simulink library "lib_S7RRRRRRR1_dynamics"  (Simulink 8.5)
settings: Solver=ode45  StartTime=0.0  StopTime=10.0  RelTol=1e-3
values from neighbouring files (symbols this model uses):
  MPV = t1    [S7RRRRRRR1_convert_par2_MPV_fixb.m]
undefined symbols (not defined in the file or in its folder): eulxyz2r, eulxyzD2omega, g_base, g_world, phi_base_t0, phiD_base_t0, pkin, q_t0, qD_t0
undefined symbols (not defined in the file): DynPar1, qJ_t0, qJD_t0, r_base_t0, rD_base_t0
libraries: lib_S7RRRRRRR1_dynamics x20, lib_transformations x8, lib_rigid_body_kinematics x6
settings Model: Creator=schappler  LastModifiedBy=schappler

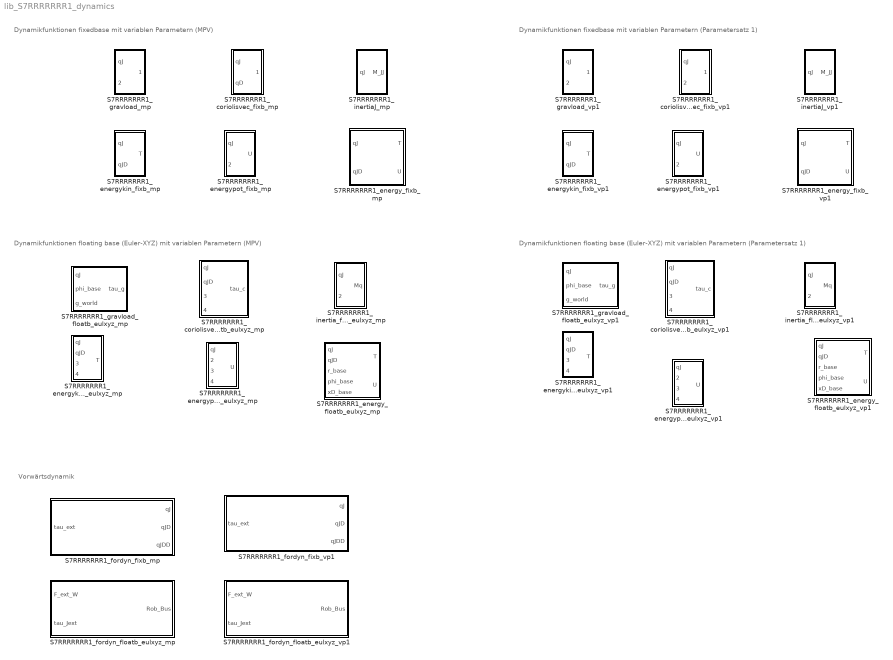
== system lib_S7RRRRRRR1_dynamics ==
  note: Vorwärtsdynamik
  note: Dynamikfunktionen fixedbase mit variablen Parametern (MPV)
  note: Dynamikfunktionen fixedbase mit variablen Parametern (Parametersatz 1)
  note: Dynamikfunktionen floating base (Euler-XYZ) mit variablen Parametern (Parametersatz 1)
  note: Dynamikfunktionen floating base (Euler-XYZ) mit variablen Parametern (MPV)
  S7RRRRRRR1_coriolisvec_fixb_mp : Subsystem  mask{pkin=pkin, MPV=MPV}
      mask prompts: pkin "Kinematik-Parameter"; MPV "Dynamik-Parameter (Minimalparametervektor fixed-base)"
      mask init:
      | NQJ=7;
  S7RRRRRRR1_coriolisvec_fixb_vp1 : Subsystem  mask{pkin=pkin, DynPar1=DynPar1}
      mask prompts: pkin "Kinematik-Parameter"; DynPar1 "Dynamik-Parameter (Parametersatz 1)"
      mask init:
      | NQJ=7;
      | m = DynPar1.m;
      | r_S = DynPar1.r_S;
      | I_S = DynPar1.I_S;
  S7RRRRRRR1_coriolisvec_floatb_eulxyz_mp : Subsystem  mask{pkin=pkin, MPV=MPV}
      mask prompts: pkin "Kinematik-Parameter"; MPV "Dynamik-Parameter (Minimalparametervektor floating-base)"
      mask init:
      | NQJ=7;
  S7RRRRRRR1_coriolisvec_floatb_eulxyz_vp1 : Subsystem  mask{pkin=pkin, DynPar1=DynPar1}
      mask prompts: pkin "Kinematik-Parameter"; DynPar1 "Dynamik-Parameter (Parametersatz 1)"
      mask init:
      | NQJ=7;
      | m = DynPar1.m;
      | r_S = DynPar1.r_S;
      | I_S = DynPar1.I_S;
  S7RRRRRRR1_energy_fixb_mp : Subsystem  mask{pkin=pkin, MPV=MPV, g_base=g_base}
      mask prompts: pkin "Kinematik-Parameter"; MPV "Dynamik-Parameter (Minimalparametervektor fixed-base)"; g_base "Gravitationsvektor im Basis-KS (g_base)"
      mask init:
      | NQJ=7;
  S7RRRRRRR1_energy_fixb_vp1 : Subsystem  mask{pkin=pkin, DynPar1=DynPar1, g_base=g_base}
      mask prompts: pkin "Kinematik-Parameter"; DynPar1 "Dynamik-Parameter (Parametersatz 1)"; g_base "Gravitationsvektor im Basis-KS (g_base)"
      mask init:
      | NQJ=7;
  S7RRRRRRR1_energy_floatb_eulxyz_mp : Subsystem  mask{pkin=pkin, MPV=MPV, g_world=g_world}
      mask prompts: pkin "Kinematik-Parameter"; MPV "Dynamik-Parameter (Minimalparametervektor floating-base)"; g_world "Gravitationsvektor im Welt-KS (g_world)"
      mask init:
      | NQJ=7;
  S7RRRRRRR1_energy_floatb_eulxyz_vp1 : Subsystem  mask{pkin=pkin, DynPar1=DynPar1, g_world=g_world}
      mask prompts: pkin "Kinematik-Parameter"; DynPar1 "Dynamik-Parameter (Parametersatz 1)"; g_world "Gravitationsvektor im Welt-KS (g_world)"
      mask init:
      | NQJ=7;
  S7RRRRRRR1_energykin_fixb_mp : Subsystem  mask{pkin=pkin, MPV=MPV}
      mask prompts: pkin "Kinematik-Parameter"; MPV "Dynamik-Parameter (Minimalparametervektor fixed-base)"
  S7RRRRRRR1_energykin_fixb_vp1 : Subsystem  mask{pkin=pkin, DynPar1=DynPar1}
      mask prompts: pkin "Kinematik-Parameter"; DynPar1 "Dynamik-Parameter (Parametersatz 1)"
      mask init:
      | NQJ=7;
      | m = DynPar1.m;
      | r_S = DynPar1.r_S;
      | I_S = DynPar1.I_S;
  S7RRRRRRR1_energykin_floatb_eulxyz_mp : Subsystem  mask{pkin=pkin, MPV=MPV}
      mask prompts: pkin "Kinematik-Parameter"; MPV "Dynamik-Parameter (Minimalparametervektor floating-base)"
      mask init:
      | NQJ=7;
  S7RRRRRRR1_energykin_floatb_eulxyz_vp1 : Subsystem  mask{pkin=pkin, DynPar1=DynPar1}
      mask prompts: pkin "Kinematik-Parameter"; DynPar1 "Dynamik-Parameter (Parametersatz 1)"
      mask init:
      | NQJ=7;
      | m = DynPar1.m;
      | r_S = DynPar1.r_S;
      | I_S = DynPar1.I_S;
  S7RRRRRRR1_energypot_fixb_mp : Subsystem  mask{pkin=pkin, MPV=MPV}
      mask prompts: pkin "Kinematik-Parameter"; MPV "Dynamik-Parameter (Minimalparametervektor fixed-base)"
      mask init:
      | NQJ=7;
  S7RRRRRRR1_energypot_fixb_vp1 : Subsystem  mask{pkin=pkin, DynPar1=DynPar1}
      mask prompts: pkin "Kinematik-Parameter"; DynPar1 "Dynamik-Parameter (Parametersatz 1)"
      mask init:
      | NQJ=7;
      | m = DynPar1.m;
      | r_S = DynPar1.r_S;
      | I_S = DynPar1.I_S;
  S7RRRRRRR1_energypot_floatb_eulxyz_mp : Subsystem  mask{pkin=pkin, MPV=MPV}
      mask prompts: pkin "Kinematik-Parameter"; MPV "Dynamik-Parameter (Minimalparametervektor floating-base)"
      mask init:
      | NQJ=7;
  S7RRRRRRR1_energypot_floatb_eulxyz_vp1 : Subsystem  mask{pkin=pkin, DynPar1=DynPar1}
      mask prompts: pkin "Kinematik-Parameter"; DynPar1 "Dynamik-Parameter (Parametersatz 1)"
      mask init:
      | NQJ=7;
      | m = DynPar1.m;
      | r_S = DynPar1.r_S;
      | I_S = DynPar1.I_S;
  S7RRRRRRR1_fordyn_fixb_mp : Subsystem  mask{q_t0=q_t0, qD_t0=qD_t0, g_base=g_base, pkin=pkin, MPV=MPV}
      mask prompts: q_t0 "q0 (initial pose)"; qD_t0 "qD0 (initial velocity)"; pkin "Kinematik-Parameter"; MPV "Dynamik-Parameter (Minimalparametervektor fixed-base)"
      mask init:
      | NQJ=7;
  S7RRRRRRR1_fordyn_fixb_vp1 : Subsystem  mask{q_t0=q_t0, qD_t0=qD_t0, g_base=g_base, pkin=pkin, DynPar1=DynPar1}
      mask prompts: q_t0 "q0 (initial pose)"; qD_t0 "qD0 (initial velocity)"; pkin "Kinematik-Parameter"; DynPar1 "Dynamik-Parameter (Parametersatz 1)"
      mask init:
      | NQJ=7;
  S7RRRRRRR1_fordyn_floatb_eulxyz_mp : Subsystem  mask{r_base_t0=r_base_t0, rD_base_t0=rD_base_t0, phi_base_t0=phi_base_t0, phiD_base_t0=phiD_base_t0, qJ_t0=qJ_t0, qJD_t0=qJD_t0, g_world=g_world, pkin=pkin, MPV=MPV}
      mask prompts: r_base_t0 "r_base_t0 (Basisposition im Welt-KS)"; qJ_t0 "q0 (initial pose)"; qJD_t0 "qD0 (initial velocity)"; pkin "Kinematik-Parameter"; MPV "Dynamik-Parameter (Minimalparametervektor floating-base)"
      mask init:
      | NQJ=7;
      mask Display:
      | port_label('input', 1, '_{(W)} F^{ext}', 'texmode', 'on')
      | port_label('input', 2, '\tau^{ext}_{J}', 'texmode', 'on')
      | port_label('output', 1, 'Rob_Bus')
  S7RRRRRRR1_fordyn_floatb_eulxyz_vp1 : Subsystem  mask{r_base_t0=r_base_t0, rD_base_t0=rD_base_t0, phi_base_t0=phi_base_t0, phiD_base_t0=phiD_base_t0, qJ_t0=qJ_t0, qJD_t0=qJD_t0, g_world=g_world, pkin=pkin, DynPar1=DynPar1}
      mask prompts: r_base_t0 "r_base_t0 (Basisposition im Welt-KS)"; qJ_t0 "q0 (initial pose)"; qJD_t0 "qD0 (initial velocity)"; pkin "Kinematik-Parameter"; DynPar1 "Dynamik-Parameter (Parametersatz 1)"
      mask init:
      | NQJ=7;
      mask Display:
      | port_label('input', 1, '_{(W)} F^{ext}', 'texmode', 'on')
      | port_label('input', 2, '\tau^{ext}_{J}', 'texmode', 'on')
      | port_label('output', 1, 'Rob_Bus')
  S7RRRRRRR1_gravload_floatb_eulxyz_mp : Subsystem  mask{pkin=pkin, MPV=MPV}
      mask prompts: pkin "Kinematik-Parameter"; MPV "Dynamik-Parameter (Minimalparametervektor floating-base)"
      mask init:
      | NQJ=7;
  S7RRRRRRR1_gravload_floatb_eulxyz_vp1 : Subsystem  mask{pkin=pkin, DynPar1=DynPar1}
      mask prompts: pkin "Kinematik-Parameter"; DynPar1 "Dynamik-Parameter (Parametersatz 1)"
      mask init:
      | NQJ=7;
      | m = DynPar1.m;
      | r_S = DynPar1.r_S;
      | I_S = DynPar1.I_S;
  S7RRRRRRR1_gravload_mp : Subsystem  mask{pkin=pkin, MPV=MPV}
      mask prompts: pkin "Kinematik-Parameter"; MPV "Dynamik-Parameter (Minimalparametervektor fixed-base)"
      mask init:
      | NQJ=7;
  S7RRRRRRR1_gravload_vp1 : Subsystem  mask{pkin=pkin, DynPar1=DynPar1}
      mask prompts: pkin "Kinematik-Parameter"; DynPar1 "Dynamik-Parameter (Parametersatz 1)"
      mask init:
      | NQJ=7;
      | m = DynPar1.m;
      | r_S = DynPar1.r_S;
      | I_S = DynPar1.I_S;
  S7RRRRRRR1_inertiaJ_mp : Subsystem  mask{pkin=pkin, MPV=MPV}
      mask prompts: pkin "Kinematik-Parameter"; MPV "Dynamik-Parameter (Minimalparametervektor fixed-base)"
      mask init:
      | NQJ=7;
  S7RRRRRRR1_inertiaJ_vp1 : Subsystem  mask{pkin=pkin, DynPar1=DynPar1}
      mask prompts: pkin "Kinematik-Parameter"; DynPar1 "Dynamik-Parameter (Parametersatz 1)"
      mask init:
      | NQJ=7;
      | m = DynPar1.m;
      | r_S = DynPar1.r_S;
      | I_S = DynPar1.I_S;
  S7RRRRRRR1_inertia_floatb_eulxyz_mp : Subsystem  mask{pkin=pkin, MPV=MPV}
      mask prompts: pkin "Kinematik-Parameter"; MPV "Dynamik-Parameter (Minimalparametervektor floating-base)"
      mask init:
      | NQJ=7;
  S7RRRRRRR1_inertia_floatb_eulxyz_vp1 : Subsystem  mask{pkin=pkin, DynPar1=DynPar1}
      mask prompts: pkin "Kinematik-Parameter"; DynPar1 "Dynamik-Parameter (Parametersatz 1)"
      mask init:
      | NQJ=7;
      | m = DynPar1.m;
      | r_S = DynPar1.r_S;
      | I_S = DynPar1.I_S;

== system lib_S7RRRRRRR1_dynamics/S7RRRRRRR1_coriolisvec_fixb_mp ==
  qJ : Inport  PortDimensions=NQJ
  qD : Inport  Port=2
  Constant5 : Constant  Value=MPV
  Constant6 : Constant  Value=pkin
  coriolisvec_fcn : MATLAB Function  TreatAsAtomicUnit=on
  tauJ_c : Outport  PortDimensions=NQJ
  wires:
  coriolisvec_fcn/1(taug) -> tauJ_c/1
  Constant6/1 -> coriolisvec_fcn/3(pkin)
  qD/1 -> coriolisvec_fcn/2(qD)
  qJ/1 -> coriolisvec_fcn/1(q)
  Constant5/1 -> coriolisvec_fcn/4(MPV)

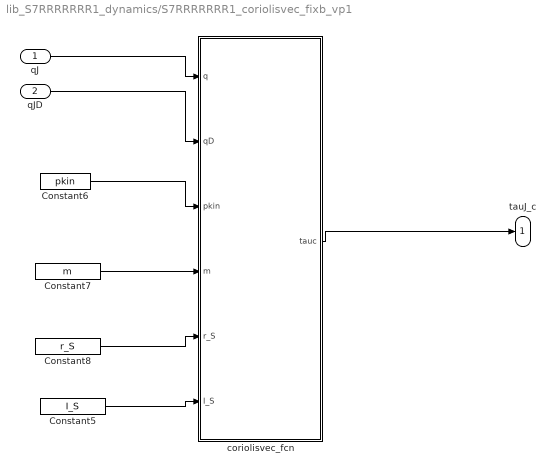
== system lib_S7RRRRRRR1_dynamics/S7RRRRRRR1_coriolisvec_fixb_vp1 ==
  qJ : Inport  PortDimensions=NQJ
  qJD : Inport  Port=2  PortDimensions=NQJ
  Constant5 : Constant  Value=I_S
  Constant6 : Constant  Value=pkin
  Constant7 : Constant  Value=m
  Constant8 : Constant  Value=r_S
  coriolisvec_fcn : MATLAB Function  TreatAsAtomicUnit=on
  tauJ_c : Outport  PortDimensions=NQJ
  wires:
  coriolisvec_fcn/1(tauc) -> tauJ_c/1
  Constant6/1 -> coriolisvec_fcn/3(pkin)
  qJD/1 -> coriolisvec_fcn/2(qD)
  qJ/1 -> coriolisvec_fcn/1(q)
  Constant7/1 -> coriolisvec_fcn/4(m)
  Constant8/1 -> coriolisvec_fcn/5(r_S)
  Constant5/1 -> coriolisvec_fcn/6(I_S)

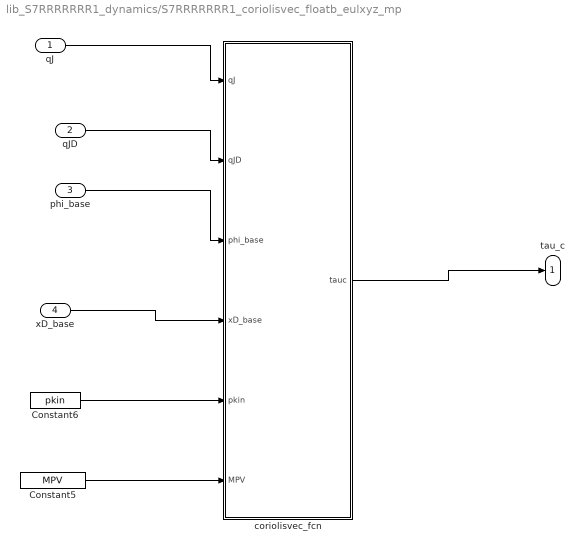
== system lib_S7RRRRRRR1_dynamics/S7RRRRRRR1_coriolisvec_floatb_eulxyz_mp ==
  qJ : Inport  PortDimensions=NQJ
  qJD : Inport  Port=2  PortDimensions=NQJ
  phi_base : Inport  Port=3  PortDimensions=3
  xD_base : Inport  Port=4  PortDimensions=6
  Constant5 : Constant  Value=MPV
  Constant6 : Constant  Value=pkin
  coriolisvec_fcn : MATLAB Function  TreatAsAtomicUnit=on
  tau_c : Outport  PortDimensions=6+NQJ
  wires:
  coriolisvec_fcn/1(tauc) -> tau_c/1
  Constant6/1 -> coriolisvec_fcn/5(pkin)
  qJD/1 -> coriolisvec_fcn/2(qJD)
  qJ/1 -> coriolisvec_fcn/1(qJ)
  Constant5/1 -> coriolisvec_fcn/6(MPV)
  phi_base/1 -> coriolisvec_fcn/3(phi_base)
  xD_base/1 -> coriolisvec_fcn/4(xD_base)

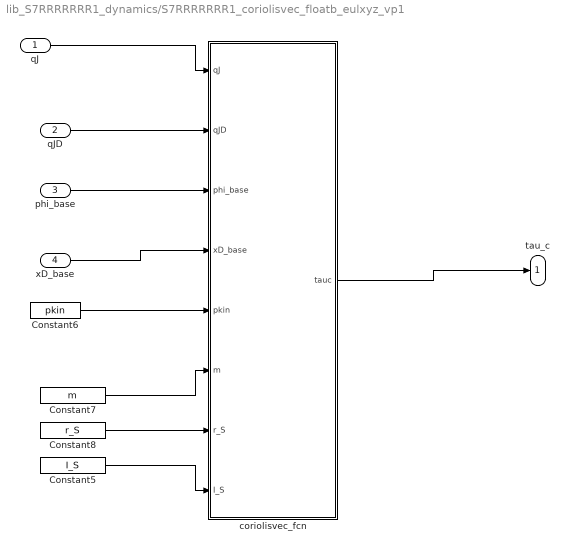
== system lib_S7RRRRRRR1_dynamics/S7RRRRRRR1_coriolisvec_floatb_eulxyz_vp1 ==
  qJ : Inport  PortDimensions=NQJ
  qJD : Inport  Port=2  PortDimensions=NQJ
  phi_base : Inport  Port=3  PortDimensions=3
  xD_base : Inport  Port=4  PortDimensions=6
  Constant5 : Constant  Value=I_S
  Constant6 : Constant  Value=pkin
  Constant7 : Constant  Value=m
  Constant8 : Constant  Value=r_S
  coriolisvec_fcn : MATLAB Function  TreatAsAtomicUnit=on
  tau_c : Outport  PortDimensions=6+NQJ
  wires:
  coriolisvec_fcn/1(tauc) -> tau_c/1
  Constant6/1 -> coriolisvec_fcn/5(pkin)
  qJD/1 -> coriolisvec_fcn/2(qJD)
  qJ/1 -> coriolisvec_fcn/1(qJ)
  Constant7/1 -> coriolisvec_fcn/6(m)
  Constant8/1 -> coriolisvec_fcn/7(r_S)
  Constant5/1 -> coriolisvec_fcn/8(I_S)
  phi_base/1 -> coriolisvec_fcn/3(phi_base)
  xD_base/1 -> coriolisvec_fcn/4(xD_base)

== system lib_S7RRRRRRR1_dynamics/S7RRRRRRR1_energy_fixb_mp ==
  qJ : Inport  PortDimensions=NQJ
  qJD : Inport  Port=2  PortDimensions=NQJ
  Constant : Constant  Value=g_base
  S7RRRRRRR1_energykin_fixb_mp : lib_S7RRRRRRR1_dynamics/S7RRRRRRR1_energykin_fixb_mp  pkin=pkin  MPV=MPV
  S7RRRRRRR1_energypot_fixb_mp : lib_S7RRRRRRR1_dynamics/S7RRRRRRR1_energypot_fixb_mp  pkin=pkin  MPV=MPV
  T : Outport  PortDimensions=1
  U : Outport  Port=2  PortDimensions=1
  wires:
  Constant/1 -> S7RRRRRRR1_energypot_fixb_mp/2
  qJD/1 -> S7RRRRRRR1_energykin_fixb_mp/2
  qJ/1 -> S7RRRRRRR1_energypot_fixb_mp/1, S7RRRRRRR1_energykin_fixb_mp/1
  S7RRRRRRR1_energypot_fixb_mp/1 -> U/1
  S7RRRRRRR1_energykin_fixb_mp/1 -> T/1

== system lib_S7RRRRRRR1_dynamics/S7RRRRRRR1_energy_fixb_vp1 ==
  qJ : Inport  PortDimensions=NQJ
  qJD : Inport  Port=2  PortDimensions=NQJ
  Constant : Constant  Value=g_base
  S7RRRRRRR1_energykin_fixb : lib_S7RRRRRRR1_dynamics/S7RRRRRRR1_energykin_fixb_vp1  pkin=pkin  DynPar1=DynPar1
  S7RRRRRRR1_energypot_fixb : lib_S7RRRRRRR1_dynamics/S7RRRRRRR1_energypot_fixb_vp1  pkin=pkin  DynPar1=DynPar1
  T : Outport  PortDimensions=1
  U : Outport  Port=2  PortDimensions=1
  wires:
  Constant/1 -> S7RRRRRRR1_energypot_fixb/2
  qJD/1 -> S7RRRRRRR1_energykin_fixb/2
  qJ/1 -> S7RRRRRRR1_energypot_fixb/1, S7RRRRRRR1_energykin_fixb/1
  S7RRRRRRR1_energypot_fixb/1 -> U/1
  S7RRRRRRR1_energykin_fixb/1 -> T/1

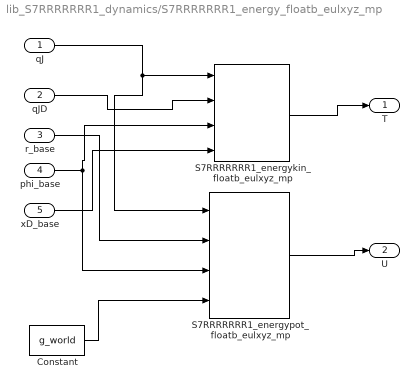
== system lib_S7RRRRRRR1_dynamics/S7RRRRRRR1_energy_floatb_eulxyz_mp ==
  qJ : Inport  PortDimensions=NQJ
  qJD : Inport  Port=2  PortDimensions=NQJ
  r_base : Inport  Port=3  PortDimensions=3
  phi_base : Inport  Port=4  PortDimensions=3
  xD_base : Inport  Port=5  PortDimensions=6
  Constant : Constant  Value=g_world
  S7RRRRRRR1_energykin_floatb_eulxyz_mp : lib_S7RRRRRRR1_dynamics/S7RRRRRRR1_energykin_floatb_eulxyz_mp  pkin=pkin  MPV=MPV
  S7RRRRRRR1_energypot_floatb_eulxyz_mp : lib_S7RRRRRRR1_dynamics/S7RRRRRRR1_energypot_floatb_eulxyz_mp  pkin=pkin  MPV=MPV
  T : Outport
  U : Outport  Port=2
  wires:
  Constant/1 -> S7RRRRRRR1_energypot_floatb_eulxyz_mp/4
  qJD/1 -> S7RRRRRRR1_energykin_floatb_eulxyz_mp/2
  qJ/1 -> S7RRRRRRR1_energypot_floatb_eulxyz_mp/1, S7RRRRRRR1_energykin_floatb_eulxyz_mp/1
  S7RRRRRRR1_energypot_floatb_eulxyz_mp/1 -> U/1
  S7RRRRRRR1_energykin_floatb_eulxyz_mp/1 -> T/1
  phi_base/1 -> S7RRRRRRR1_energypot_floatb_eulxyz_mp/3, S7RRRRRRR1_energykin_floatb_eulxyz_mp/3
  r_base/1 -> S7RRRRRRR1_energypot_floatb_eulxyz_mp/2
  xD_base/1 -> S7RRRRRRR1_energykin_floatb_eulxyz_mp/4

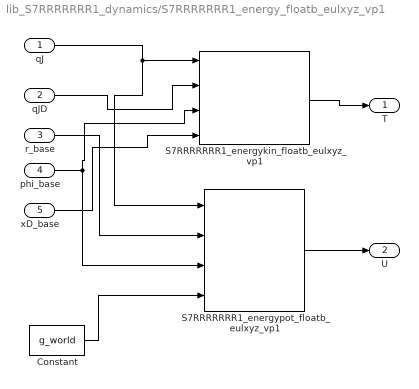
== system lib_S7RRRRRRR1_dynamics/S7RRRRRRR1_energy_floatb_eulxyz_vp1 ==
  qJ : Inport  PortDimensions=NQJ
  qJD : Inport  Port=2  PortDimensions=NQJ
  r_base : Inport  Port=3  PortDimensions=3
  phi_base : Inport  Port=4  PortDimensions=3
  xD_base : Inport  Port=5  PortDimensions=6
  Constant : Constant  Value=g_world
  S7RRRRRRR1_energykin_floatb_eulxyz_vp1 : lib_S7RRRRRRR1_dynamics/S7RRRRRRR1_energykin_floatb_eulxyz_vp1  pkin=pkin  DynPar1=DynPar1
  S7RRRRRRR1_energypot_floatb_eulxyz_vp1 : lib_S7RRRRRRR1_dynamics/S7RRRRRRR1_energypot_floatb_eulxyz_vp1  pkin=pkin  DynPar1=DynPar1
  T : Outport
  U : Outport  Port=2
  wires:
  Constant/1 -> S7RRRRRRR1_energypot_floatb_eulxyz_vp1/4
  qJD/1 -> S7RRRRRRR1_energykin_floatb_eulxyz_vp1/2
  qJ/1 -> S7RRRRRRR1_energypot_floatb_eulxyz_vp1/1, S7RRRRRRR1_energykin_floatb_eulxyz_vp1/1
  S7RRRRRRR1_energypot_floatb_eulxyz_vp1/1 -> U/1
  S7RRRRRRR1_energykin_floatb_eulxyz_vp1/1 -> T/1
  phi_base/1 -> S7RRRRRRR1_energykin_floatb_eulxyz_vp1/3, S7RRRRRRR1_energypot_floatb_eulxyz_vp1/3
  r_base/1 -> S7RRRRRRR1_energypot_floatb_eulxyz_vp1/2
  xD_base/1 -> S7RRRRRRR1_energykin_floatb_eulxyz_vp1/4

== system lib_S7RRRRRRR1_dynamics/S7RRRRRRR1_energykin_fixb_mp ==
  qJ : Inport  PortDimensions=NQJ
  qJD : Inport  Port=2  PortDimensions=NQJ
  Constant5 : Constant  Value=MPV
  Constant6 : Constant  Value=pkin
  energykin_fcn : MATLAB Function  TreatAsAtomicUnit=on
  T : Outport  PortDimensions=1
  wires:
  energykin_fcn/1(T) -> T/1
  Constant6/1 -> energykin_fcn/3(pkin)
  qJD/1 -> energykin_fcn/2(qD)
  qJ/1 -> energykin_fcn/1(q)
  Constant5/1 -> energykin_fcn/4(MPV)

== system lib_S7RRRRRRR1_dynamics/S7RRRRRRR1_energykin_fixb_vp1 ==
  qJ : Inport  PortDimensions=NQJ
  qJD : Inport  Port=2  PortDimensions=NQJ
  Constant5 : Constant  Value=I_S
  Constant6 : Constant  Value=pkin
  Constant7 : Constant  Value=m
  Constant8 : Constant  Value=r_S
  MATLAB Function : MATLAB Function  TreatAsAtomicUnit=on
  T : Outport
  wires:
  MATLAB Function/1(T) -> T/1
  Constant6/1 -> MATLAB Function/3(pkin)
  qJD/1 -> MATLAB Function/2(qD)
  qJ/1 -> MATLAB Function/1(q)
  Constant7/1 -> MATLAB Function/4(m)
  Constant8/1 -> MATLAB Function/5(r_S)
  Constant5/1 -> MATLAB Function/6(I_S)

== system lib_S7RRRRRRR1_dynamics/S7RRRRRRR1_energykin_floatb_eulxyz_mp ==
  qJ : Inport  PortDimensions=NQJ
  qJD : Inport  Port=2  PortDimensions=NQJ
  phi_base : Inport  Port=3  PortDimensions=3
  xD_base : Inport  Port=4  PortDimensions=6
  Constant1 : Constant  Value=MPV
  Constant6 : Constant  Value=pkin
  MATLAB Function : MATLAB Function  TreatAsAtomicUnit=on
  T : Outport  PortDimensions=1
  wires:
  MATLAB Function/1(T) -> T/1
  Constant6/1 -> MATLAB Function/5(pkin)
  qJD/1 -> MATLAB Function/2(qD)
  qJ/1 -> MATLAB Function/1(qJ)
  Constant1/1 -> MATLAB Function/6(MPV)
  phi_base/1 -> MATLAB Function/3(phi_base)
  xD_base/1 -> MATLAB Function/4(xD_base)

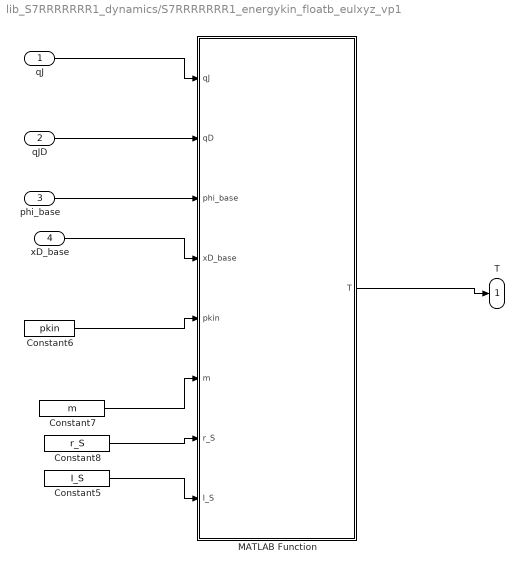
== system lib_S7RRRRRRR1_dynamics/S7RRRRRRR1_energykin_floatb_eulxyz_vp1 ==
  qJ : Inport  PortDimensions=NQJ
  qJD : Inport  Port=2  PortDimensions=NQJ
  phi_base : Inport  Port=3  PortDimensions=3
  xD_base : Inport  Port=4  PortDimensions=6
  Constant5 : Constant  Value=I_S
  Constant6 : Constant  Value=pkin
  Constant7 : Constant  Value=m
  Constant8 : Constant  Value=r_S
  MATLAB Function : MATLAB Function  TreatAsAtomicUnit=on
  T : Outport  PortDimensions=1
  wires:
  MATLAB Function/1(T) -> T/1
  Constant6/1 -> MATLAB Function/5(pkin)
  qJD/1 -> MATLAB Function/2(qD)
  qJ/1 -> MATLAB Function/1(qJ)
  Constant7/1 -> MATLAB Function/6(m)
  Constant8/1 -> MATLAB Function/7(r_S)
  Constant5/1 -> MATLAB Function/8(I_S)
  phi_base/1 -> MATLAB Function/3(phi_base)
  xD_base/1 -> MATLAB Function/4(xD_base)

== system lib_S7RRRRRRR1_dynamics/S7RRRRRRR1_energypot_fixb_mp ==
  qJ : Inport  PortDimensions=NQJ
  g_base : Inport  Port=2
  Constant5 : Constant  Value=MPV
  Constant6 : Constant  Value=pkin
  energypot_fcn : MATLAB Function  TreatAsAtomicUnit=on
  U : Outport  PortDimensions=1
  wires:
  energypot_fcn/1(T) -> U/1
  Constant6/1 -> energypot_fcn/3(pkin)
  g_base/1 -> energypot_fcn/2(g_base)
  qJ/1 -> energypot_fcn/1(q)
  Constant5/1 -> energypot_fcn/4(MPV)

== system lib_S7RRRRRRR1_dynamics/S7RRRRRRR1_energypot_fixb_vp1 ==
  qJ : Inport  PortDimensions=NQJ
  g_base : Inport  Port=2  PortDimensions=3
  Constant6 : Constant  Value=pkin
  Constant7 : Constant  Value=m
  Constant8 : Constant  Value=r_S
  MATLAB Function : MATLAB Function  TreatAsAtomicUnit=on
  U : Outport
  wires:
  MATLAB Function/1(U) -> U/1
  Constant6/1 -> MATLAB Function/3(pkin)
  g_base/1 -> MATLAB Function/2(g_base)
  qJ/1 -> MATLAB Function/1(q)
  Constant7/1 -> MATLAB Function/4(m)
  Constant8/1 -> MATLAB Function/5(r_S)

== system lib_S7RRRRRRR1_dynamics/S7RRRRRRR1_energypot_floatb_eulxyz_mp ==
  qJ : Inport  PortDimensions=NQJ
  r_base : Inport  Port=2  PortDimensions=3
  phi_base : Inport  Port=3  PortDimensions=3
  g_world : Inport  Port=4  PortDimensions=3
  Constant5 : Constant  Value=MPV
  Constant6 : Constant  Value=pkin
  MATLAB Function : MATLAB Function  TreatAsAtomicUnit=on
  U : Outport
  wires:
  MATLAB Function/1(U) -> U/1
  Constant6/1 -> MATLAB Function/5(pkin)
  g_world/1 -> MATLAB Function/4(g_world)
  qJ/1 -> MATLAB Function/1(qJ)
  r_base/1 -> MATLAB Function/2(r_base)
  phi_base/1 -> MATLAB Function/3(phi_base)
  Constant5/1 -> MATLAB Function/6(MPV)

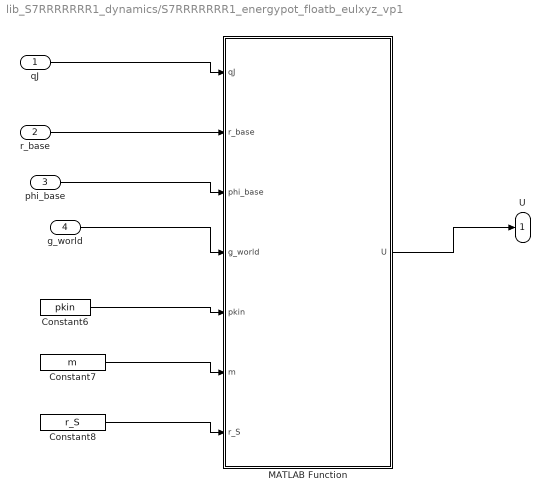
== system lib_S7RRRRRRR1_dynamics/S7RRRRRRR1_energypot_floatb_eulxyz_vp1 ==
  qJ : Inport  PortDimensions=NQJ
  r_base : Inport  Port=2  PortDimensions=3
  phi_base : Inport  Port=3  PortDimensions=3
  g_world : Inport  Port=4  PortDimensions=3
  Constant6 : Constant  Value=pkin
  Constant7 : Constant  Value=m
  Constant8 : Constant  Value=r_S
  MATLAB Function : MATLAB Function  TreatAsAtomicUnit=on
  U : Outport
  wires:
  MATLAB Function/1(U) -> U/1
  Constant6/1 -> MATLAB Function/5(pkin)
  g_world/1 -> MATLAB Function/4(g_world)
  qJ/1 -> MATLAB Function/1(qJ)
  Constant7/1 -> MATLAB Function/6(m)
  Constant8/1 -> MATLAB Function/7(r_S)
  r_base/1 -> MATLAB Function/2(r_base)
  phi_base/1 -> MATLAB Function/3(phi_base)

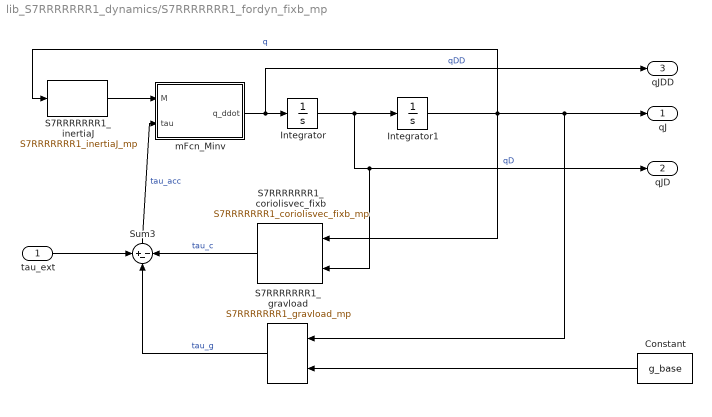
== system lib_S7RRRRRRR1_dynamics/S7RRRRRRR1_fordyn_fixb_mp ==
  "tau_ext " : Inport  PortDimensions=NQJ
  Constant : Constant  Value=g_base
  Integrator : Integrator  InitialCondition=qD_t0
  Integrator1 : Integrator  InitialCondition=q_t0
  Sum3 : Sum  Inputs=+--
  S7RRRRRRR1_coriolisvec_fixb : lib_S7RRRRRRR1_dynamics/S7RRRRRRR1_coriolisvec_fixb_mp  pkin=pkin  MPV=MPV
  S7RRRRRRR1_gravload : lib_S7RRRRRRR1_dynamics/S7RRRRRRR1_gravload_mp  pkin=pkin  MPV=MPV
  S7RRRRRRR1_inertiaJ : lib_S7RRRRRRR1_dynamics/S7RRRRRRR1_inertiaJ_mp  pkin=pkin  MPV=MPV
  mFcn_Minv : MATLAB Function  TreatAsAtomicUnit=on
  qJ : Outport  PortDimensions=NQJ
  qJD : Outport  Port=2  PortDimensions=NQJ
  qJDD : Outport  Port=3  PortDimensions=NQJ
  wires:
  S7RRRRRRR1_gravload/1 -> Sum3/2  "tau_g"
  Integrator1/1 -> S7RRRRRRR1_coriolisvec_fixb/1, S7RRRRRRR1_inertiaJ/1, S7RRRRRRR1_gravload/1, qJ/1  "q"
  mFcn_Minv/1(q_ddot) -> qJDD/1, Integrator/1  "qDD"
  S7RRRRRRR1_coriolisvec_fixb/1 -> Sum3/3  "tau_c"
  "tau_ext "/1 -> Sum3/1
  Integrator/1 -> S7RRRRRRR1_coriolisvec_fixb/2, qJD/1, Integrator1/1  "qD"
  Sum3/1 -> mFcn_Minv/2(tau)  "tau_acc"
  S7RRRRRRR1_inertiaJ/1 -> mFcn_Minv/1(M)
  Constant/1 -> S7RRRRRRR1_gravload/2

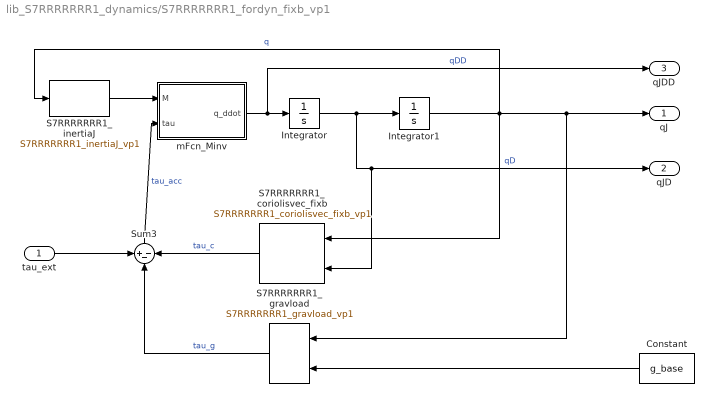
== system lib_S7RRRRRRR1_dynamics/S7RRRRRRR1_fordyn_fixb_vp1 ==
  "tau_ext " : Inport  PortDimensions=NQJ
  Constant : Constant  Value=g_base
  Integrator : Integrator  InitialCondition=qD_t0
  Integrator1 : Integrator  InitialCondition=q_t0
  Sum3 : Sum  Inputs=+--
  S7RRRRRRR1_coriolisvec_fixb : lib_S7RRRRRRR1_dynamics/S7RRRRRRR1_coriolisvec_fixb_vp1  pkin=pkin  DynPar1=DynPar1
  S7RRRRRRR1_gravload : lib_S7RRRRRRR1_dynamics/S7RRRRRRR1_gravload_vp1  pkin=pkin  DynPar1=DynPar1
  S7RRRRRRR1_inertiaJ : lib_S7RRRRRRR1_dynamics/S7RRRRRRR1_inertiaJ_vp1  pkin=pkin  DynPar1=DynPar1
  mFcn_Minv : MATLAB Function  TreatAsAtomicUnit=on
  qJ : Outport  PortDimensions=NQJ
  qJD : Outport  Port=2  PortDimensions=NQJ
  qJDD : Outport  Port=3  PortDimensions=NQJ
  wires:
  S7RRRRRRR1_gravload/1 -> Sum3/2  "tau_g"
  Integrator1/1 -> S7RRRRRRR1_coriolisvec_fixb/1, S7RRRRRRR1_inertiaJ/1, S7RRRRRRR1_gravload/1, qJ/1  "q"
  mFcn_Minv/1(q_ddot) -> qJDD/1, Integrator/1  "qDD"
  S7RRRRRRR1_coriolisvec_fixb/1 -> Sum3/3  "tau_c"
  "tau_ext "/1 -> Sum3/1
  Integrator/1 -> S7RRRRRRR1_coriolisvec_fixb/2, qJD/1, Integrator1/1  "qD"
  Sum3/1 -> mFcn_Minv/2(tau)  "tau_acc"
  S7RRRRRRR1_inertiaJ/1 -> mFcn_Minv/1(M)
  Constant/1 -> S7RRRRRRR1_gravload/2

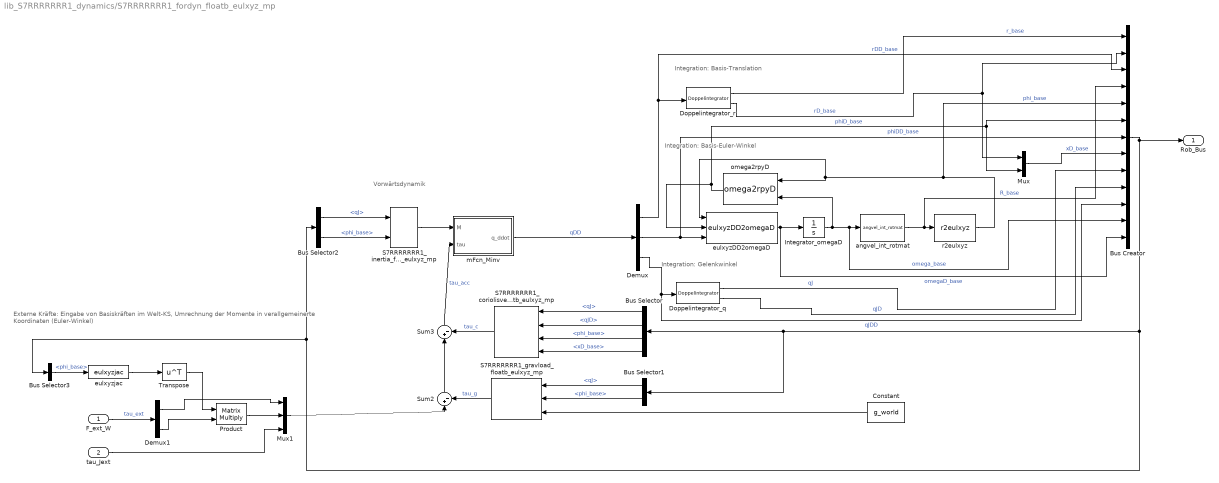
== system lib_S7RRRRRRR1_dynamics/S7RRRRRRR1_fordyn_floatb_eulxyz_mp ==
  note: Integration: Basis-Translation
  note: Integration: Gelenkwinkel
  note: Vorwärtsdynamik
  note: Integration: Basis-Euler-Winkel
  note: Externe Kräfte: Eingabe von Basiskräften im Welt-KS, Umrechnung der Momente
      | in verallgemeinerte Koordinaten (Euler-Winkel)
  F_ext_W : Inport  PortDimensions=6
  tau_Jext : Inport  Port=2  PortDimensions=NQJ
  Bus Creator : BusCreator  Inputs=13
  Bus Selector : BusSelector  OutputSignals=qJ,qJD,phi_base,xD_base
  Bus Selector1 : BusSelector  OutputSignals=qJ,phi_base
  Bus Selector2 : BusSelector  OutputSignals=qJ,phi_base
  Bus Selector3 : BusSelector  OutputSignals=phi_base
  Constant : Constant  Value=g_world
  Demux : Demux  Outputs=[3 3 NQJ]
  Demux1 : Demux  Outputs=[3 3]
  Doppelintegrator_q : lib_rigid_body_kinematics/Doppelintegrator  r0=qJ_t0  rD0=qJD_t0  Name_v='q'
  Doppelintegrator_r : lib_rigid_body_kinematics/Doppelintegrator  r0=r_base_t0  rD0=rD_base_t0  Name_v='r'
  Integrator_omegaD : Integrator  InitialCondition=eulxyzD2omega(phi_base_t0, phiD_base_t0)
  Mux : Mux  Inputs=2
  Mux1 : Mux  Inputs=[3 3 NQJ]
  Product : Product  Multiplication=Matrix(*)
  r2eulxyz : lib_transformations/r2eulxyz
  Sum2 : Sum  Inputs=|+-
  Sum3 : Sum  Inputs=|+-
  Transpose : Math  Operator=transpose  SaturateOnIntegerOverflow=on
  angvel_int_rotmat : lib_rigid_body_kinematics/angvel_int_rotmat  R_0E_t0=eulxyz2r(phi_base_t0)
  eulxyzjac : lib_transformations/eulxyzjac
  S7RRRRRRR1_coriolisvec_floatb_eulxyz_mp : lib_S7RRRRRRR1_dynamics/S7RRRRRRR1_coriolisvec_floatb_eulxyz_mp  pkin=pkin  MPV=MPV
  S7RRRRRRR1_gravload_floatb_eulxyz_mp : lib_S7RRRRRRR1_dynamics/S7RRRRRRR1_gravload_floatb_eulxyz_mp  pkin=pkin  MPV=MPV
  S7RRRRRRR1_inertia_floatb_eulxyz_mp : lib_S7RRRRRRR1_dynamics/S7RRRRRRR1_inertia_floatb_eulxyz_mp  pkin=pkin  MPV=MPV
  mFcn_Minv : MATLAB Function  TreatAsAtomicUnit=on
  omega2rpyD : lib_transformations/omega2rpyD
  eulxyzDD2omegaD : lib_transformations/eulxyzDD2omegaD
  Rob_Bus : Outport
  wires:
  Constant/1 -> S7RRRRRRR1_gravload_floatb_eulxyz_mp/3
  F_ext_W/1 -> Demux1/1  "tau_ext"
  S7RRRRRRR1_inertia_floatb_eulxyz_mp/1 -> mFcn_Minv/1(M)
  Sum3/1 -> mFcn_Minv/2(tau)  "tau_acc"
  S7RRRRRRR1_coriolisvec_floatb_eulxyz_mp/1 -> Sum3/2  "tau_c"
  Sum2/1 -> Sum3/1
  mFcn_Minv/1(q_ddot) -> Demux/1  "qDD"
  S7RRRRRRR1_gravload_floatb_eulxyz_mp/1 -> Sum2/2  "tau_g"
  Demux/1 -> Doppelintegrator_r/1, Bus Creator/3  "rDD_base"
  Demux/3 -> Bus Creator/11, Doppelintegrator_q/1  "qJDD"
  eulxyzDD2omegaD/1 -> Bus Creator/13, Integrator_omegaD/1  "omegaD_base"
  Integrator_omegaD/1 -> Bus Creator/12, angvel_int_rotmat/1, omega2rpyD/2  "omega_base"
  Demux/2 -> Bus Creator/7, eulxyzDD2omegaD/3  "phiDD_base"
  angvel_int_rotmat/1 -> Bus Creator/4, r2eulxyz/1  "R_base"
  r2eulxyz/1 -> Bus Creator/5, eulxyzDD2omegaD/1, omega2rpyD/1  "phi_base"
  omega2rpyD/1 -> eulxyzDD2omegaD/2, Mux/2, Bus Creator/6  "phiD_base"
  Doppelintegrator_r/1 -> Bus Creator/1  "r_base"
  Doppelintegrator_r/2 -> Mux/1, Bus Creator/2  "rD_base"
  Mux/1 -> Bus Creator/8  "xD_base"
  Doppelintegrator_q/1 -> Bus Creator/9  "qJ"
  Doppelintegrator_q/2 -> Bus Creator/10  "qJD"
  Bus Selector/4 -> S7RRRRRRR1_coriolisvec_floatb_eulxyz_mp/4  "<xD_base>"
  Bus Selector/3 -> S7RRRRRRR1_coriolisvec_floatb_eulxyz_mp/3  "<phi_base>"
  Bus Selector/2 -> S7RRRRRRR1_coriolisvec_floatb_eulxyz_mp/2  "<qJD>"
  Bus Selector/1 -> S7RRRRRRR1_coriolisvec_floatb_eulxyz_mp/1  "<qJ>"
  Bus Selector1/1 -> S7RRRRRRR1_gravload_floatb_eulxyz_mp/1  "<qJ>"
  Bus Selector1/2 -> S7RRRRRRR1_gravload_floatb_eulxyz_mp/2  "<phi_base>"
  Bus Selector2/1 -> S7RRRRRRR1_inertia_floatb_eulxyz_mp/1  "<qJ>"
  Bus Selector2/2 -> S7RRRRRRR1_inertia_floatb_eulxyz_mp/2  "<phi_base>"
  Bus Creator/1 -> Bus Selector2/1, Bus Selector3/1, Bus Selector1/1, Bus Selector/1, Rob_Bus/1
  Demux1/2 -> Product/2
  Bus Selector3/1 -> eulxyzjac/1  "<phi_base>"
  eulxyzjac/1 -> Transpose/1
  Product/1 -> Mux1/2
  Transpose/1 -> Product/1
  Demux1/1 -> Mux1/1
  tau_Jext/1 -> Mux1/3
  Mux1/1 -> Sum2/1

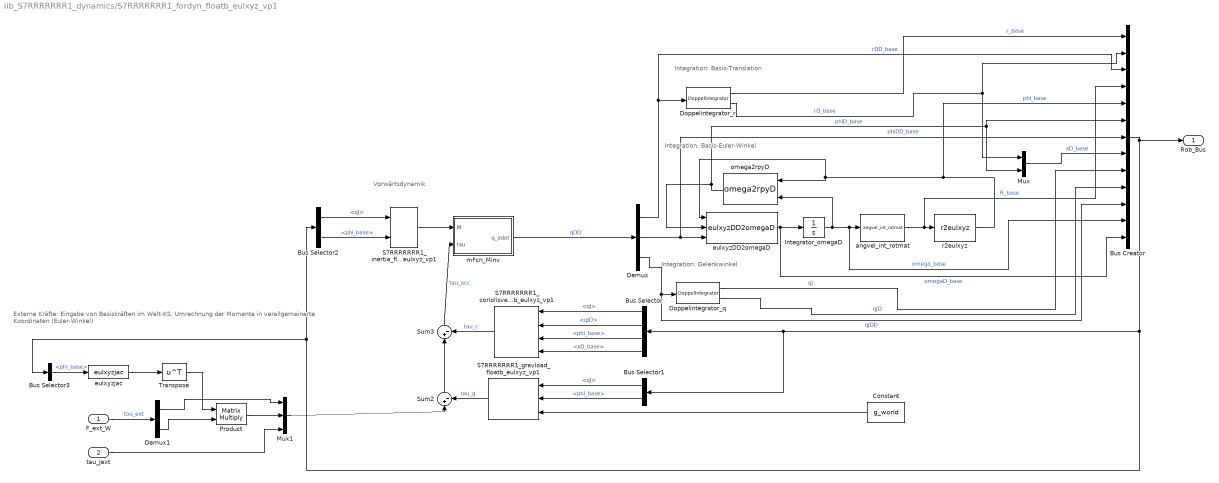
== system lib_S7RRRRRRR1_dynamics/S7RRRRRRR1_fordyn_floatb_eulxyz_vp1 ==
  note: Integration: Basis-Translation
  note: Integration: Gelenkwinkel
  note: Vorwärtsdynamik
  note: Integration: Basis-Euler-Winkel
  note: Externe Kräfte: Eingabe von Basiskräften im Welt-KS, Umrechnung der Momente
      | in verallgemeinerte Koordinaten (Euler-Winkel)
  F_ext_W : Inport  PortDimensions=6
  tau_Jext : Inport  Port=2  PortDimensions=NQJ
  Bus Creator : BusCreator  Inputs=13
  Bus Selector : BusSelector  OutputSignals=qJ,qJD,phi_base,xD_base
  Bus Selector1 : BusSelector  OutputSignals=qJ,phi_base
  Bus Selector2 : BusSelector  OutputSignals=qJ,phi_base
  Bus Selector3 : BusSelector  OutputSignals=phi_base
  Constant : Constant  Value=g_world
  Demux : Demux  Outputs=[3 3 NQJ]
  Demux1 : Demux  Outputs=[3 3]
  Doppelintegrator_q : lib_rigid_body_kinematics/Doppelintegrator  r0=qJ_t0  rD0=qJD_t0  Name_v='q'
  Doppelintegrator_r : lib_rigid_body_kinematics/Doppelintegrator  r0=r_base_t0  rD0=rD_base_t0  Name_v='r'
  Integrator_omegaD : Integrator  InitialCondition=eulxyzD2omega(phi_base_t0, phiD_base_t0)
  Mux : Mux  Inputs=2
  Mux1 : Mux  Inputs=[3 3 NQJ]
  Product : Product  Multiplication=Matrix(*)
  r2eulxyz : lib_transformations/r2eulxyz
  Sum2 : Sum  Inputs=|+-
  Sum3 : Sum  Inputs=|+-
  Transpose : Math  Operator=transpose  SaturateOnIntegerOverflow=on
  angvel_int_rotmat : lib_rigid_body_kinematics/angvel_int_rotmat  R_0E_t0=eulxyz2r(phi_base_t0)
  eulxyzjac : lib_transformations/eulxyzjac
  S7RRRRRRR1_coriolisvec_floatb_eulxyz_vp1 : lib_S7RRRRRRR1_dynamics/S7RRRRRRR1_coriolisvec_floatb_eulxyz_vp1  pkin=pkin  DynPar1=DynPar1
  S7RRRRRRR1_gravload_floatb_eulxyz_vp1 : lib_S7RRRRRRR1_dynamics/S7RRRRRRR1_gravload_floatb_eulxyz_vp1  pkin=pkin  DynPar1=DynPar1
  S7RRRRRRR1_inertia_floatb_eulxyz_vp1 : lib_S7RRRRRRR1_dynamics/S7RRRRRRR1_inertia_floatb_eulxyz_vp1  pkin=pkin  DynPar1=DynPar1
  mFcn_Minv : MATLAB Function  TreatAsAtomicUnit=on
  omega2rpyD : lib_transformations/omega2rpyD
  eulxyzDD2omegaD : lib_transformations/eulxyzDD2omegaD
  Rob_Bus : Outport
  wires:
  Constant/1 -> S7RRRRRRR1_gravload_floatb_eulxyz_vp1/3
  F_ext_W/1 -> Demux1/1  "tau_ext"
  S7RRRRRRR1_inertia_floatb_eulxyz_vp1/1 -> mFcn_Minv/1(M)
  Sum3/1 -> mFcn_Minv/2(tau)  "tau_acc"
  S7RRRRRRR1_coriolisvec_floatb_eulxyz_vp1/1 -> Sum3/2  "tau_c"
  Sum2/1 -> Sum3/1
  mFcn_Minv/1(q_ddot) -> Demux/1  "qDD"
  S7RRRRRRR1_gravload_floatb_eulxyz_vp1/1 -> Sum2/2  "tau_g"
  Demux/1 -> Doppelintegrator_r/1, Bus Creator/3  "rDD_base"
  Demux/3 -> Bus Creator/11, Doppelintegrator_q/1  "qJDD"
  eulxyzDD2omegaD/1 -> Bus Creator/13, Integrator_omegaD/1  "omegaD_base"
  Integrator_omegaD/1 -> Bus Creator/12, angvel_int_rotmat/1, omega2rpyD/2  "omega_base"
  Demux/2 -> Bus Creator/7, eulxyzDD2omegaD/3  "phiDD_base"
  angvel_int_rotmat/1 -> Bus Creator/4, r2eulxyz/1  "R_base"
  r2eulxyz/1 -> Bus Creator/5, eulxyzDD2omegaD/1, omega2rpyD/1  "phi_base"
  omega2rpyD/1 -> eulxyzDD2omegaD/2, Mux/2, Bus Creator/6  "phiD_base"
  Doppelintegrator_r/1 -> Bus Creator/1  "r_base"
  Doppelintegrator_r/2 -> Mux/1, Bus Creator/2  "rD_base"
  Mux/1 -> Bus Creator/8  "xD_base"
  Doppelintegrator_q/1 -> Bus Creator/9  "qJ"
  Doppelintegrator_q/2 -> Bus Creator/10  "qJD"
  Bus Selector/4 -> S7RRRRRRR1_coriolisvec_floatb_eulxyz_vp1/4  "<xD_base>"
  Bus Selector/3 -> S7RRRRRRR1_coriolisvec_floatb_eulxyz_vp1/3  "<phi_base>"
  Bus Selector/2 -> S7RRRRRRR1_coriolisvec_floatb_eulxyz_vp1/2  "<qJD>"
  Bus Selector/1 -> S7RRRRRRR1_coriolisvec_floatb_eulxyz_vp1/1  "<qJ>"
  Bus Selector1/1 -> S7RRRRRRR1_gravload_floatb_eulxyz_vp1/1  "<qJ>"
  Bus Selector1/2 -> S7RRRRRRR1_gravload_floatb_eulxyz_vp1/2  "<phi_base>"
  Bus Selector2/1 -> S7RRRRRRR1_inertia_floatb_eulxyz_vp1/1  "<qJ>"
  Bus Selector2/2 -> S7RRRRRRR1_inertia_floatb_eulxyz_vp1/2  "<phi_base>"
  Bus Creator/1 -> Bus Selector2/1, Bus Selector3/1, Bus Selector1/1, Bus Selector/1, Rob_Bus/1
  Demux1/2 -> Product/2
  Bus Selector3/1 -> eulxyzjac/1  "<phi_base>"
  eulxyzjac/1 -> Transpose/1
  Product/1 -> Mux1/2
  Transpose/1 -> Product/1
  Demux1/1 -> Mux1/1
  tau_Jext/1 -> Mux1/3
  Mux1/1 -> Sum2/1

== system lib_S7RRRRRRR1_dynamics/S7RRRRRRR1_gravload_floatb_eulxyz_mp ==
  qJ : Inport  PortDimensions=NQJ
  phi_base : Inport  Port=2  PortDimensions=3
  g_world : Inport  Port=3  PortDimensions=3
  Constant1 : Constant  Value=MPV
  Constant6 : Constant  Value=pkin
  MATLAB Function : MATLAB Function  TreatAsAtomicUnit=on
  tau_g : Outport  PortDimensions=6+NQJ
  wires:
  MATLAB Function/1(taug) -> tau_g/1
  Constant6/1 -> MATLAB Function/4(pkin)
  g_world/1 -> MATLAB Function/3(g_world)
  qJ/1 -> MATLAB Function/1(q)
  Constant1/1 -> MATLAB Function/5(MPV)
  phi_base/1 -> MATLAB Function/2(ob)

== system lib_S7RRRRRRR1_dynamics/S7RRRRRRR1_gravload_floatb_eulxyz_vp1 ==
  qJ : Inport  PortDimensions=NQJ
  phi_base : Inport  Port=2  PortDimensions=3
  g_world : Inport  Port=3  PortDimensions=3
  Constant5 : Constant  Value=m
  Constant6 : Constant  Value=pkin
  Constant7 : Constant  Value=r_S
  MATLAB Function : MATLAB Function  TreatAsAtomicUnit=on
  tau_g : Outport  PortDimensions=6+NQJ
  wires:
  MATLAB Function/1(taug) -> tau_g/1
  Constant6/1 -> MATLAB Function/4(pkin)
  g_world/1 -> MATLAB Function/3(g_world)
  qJ/1 -> MATLAB Function/1(q)
  Constant5/1 -> MATLAB Function/5(m)
  Constant7/1 -> MATLAB Function/6(r_S)
  phi_base/1 -> MATLAB Function/2(ob)

== system lib_S7RRRRRRR1_dynamics/S7RRRRRRR1_gravload_mp ==
  qJ : Inport  PortDimensions=NQJ
  g_base : Inport  Port=2
  Constant5 : Constant  Value=MPV
  Constant6 : Constant  Value=pkin
  gravload_Fcn : MATLAB Function  TreatAsAtomicUnit=on
  tauJ_g : Outport  PortDimensions=NQJ
  wires:
  gravload_Fcn/1(taug) -> tauJ_g/1
  Constant6/1 -> gravload_Fcn/3(pkin)
  g_base/1 -> gravload_Fcn/2(g_base)
  qJ/1 -> gravload_Fcn/1(q)
  Constant5/1 -> gravload_Fcn/4(MPV)

== system lib_S7RRRRRRR1_dynamics/S7RRRRRRR1_gravload_vp1 ==
  qJ : Inport  PortDimensions=NQJ
  g_base : Inport  Port=2  PortDimensions=3
  Constant5 : Constant  Value=m
  Constant6 : Constant  Value=pkin
  Constant7 : Constant  Value=r_S
  MATLAB Function : MATLAB Function  TreatAsAtomicUnit=on
  tau_g : Outport  PortDimensions=NQJ
  wires:
  MATLAB Function/1(taug) -> tau_g/1
  Constant6/1 -> MATLAB Function/3(pkin)
  g_base/1 -> MATLAB Function/2(g_base)
  qJ/1 -> MATLAB Function/1(q)
  Constant5/1 -> MATLAB Function/4(m)
  Constant7/1 -> MATLAB Function/5(r_S)

== system lib_S7RRRRRRR1_dynamics/S7RRRRRRR1_inertiaJ_mp ==
  qJ : Inport  PortDimensions=NQJ
  Constant5 : Constant  Value=MPV
  Constant6 : Constant  Value=pkin
  inertia_fcn : MATLAB Function  TreatAsAtomicUnit=on
  M_JJ : Outport  PortDimensions=[NQJ NQJ]
  wires:
  inertia_fcn/1(Mq) -> M_JJ/1
  Constant6/1 -> inertia_fcn/2(pkin)
  qJ/1 -> inertia_fcn/1(q)
  Constant5/1 -> inertia_fcn/3(MPV)

== system lib_S7RRRRRRR1_dynamics/S7RRRRRRR1_inertiaJ_vp1 ==
  qJ : Inport  PortDimensions=NQJ
  Constant6 : Constant  Value=pkin
  Constant7 : Constant  Value=m
  Constant8 : Constant  Value=r_S
  Constant9 : Constant  Value=I_S
  inertiajoint_fcn : MATLAB Function  TreatAsAtomicUnit=on
  M_JJ : Outport  PortDimensions=[NQJ NQJ]
  wires:
  inertiajoint_fcn/1(Mq) -> M_JJ/1
  Constant6/1 -> inertiajoint_fcn/2(pkin)
  qJ/1 -> inertiajoint_fcn/1(q)
  Constant7/1 -> inertiajoint_fcn/3(m)
  Constant8/1 -> inertiajoint_fcn/4(r_S)
  Constant9/1 -> inertiajoint_fcn/5(I_S)

== system lib_S7RRRRRRR1_dynamics/S7RRRRRRR1_inertia_floatb_eulxyz_mp ==
  qJ : Inport  PortDimensions=NQJ
  phi_base : Inport  Port=2  PortDimensions=3
  Constant5 : Constant  Value=MPV
  Constant6 : Constant  Value=pkin
  inertiajoint_fcn : MATLAB Function  TreatAsAtomicUnit=on
  Mq : Outport  PortDimensions=[6+NQJ 6+NQJ]
  wires:
  inertiajoint_fcn/1(Mq) -> Mq/1
  Constant6/1 -> inertiajoint_fcn/3(pkin)
  qJ/1 -> inertiajoint_fcn/1(qJ)
  Constant5/1 -> inertiajoint_fcn/4(MPV)
  phi_base/1 -> inertiajoint_fcn/2(phi_base)

== system lib_S7RRRRRRR1_dynamics/S7RRRRRRR1_inertia_floatb_eulxyz_vp1 ==
  qJ : Inport  PortDimensions=NQJ
  phi_base : Inport  Port=2  PortDimensions=3
  Constant6 : Constant  Value=pkin
  Constant7 : Constant  Value=m
  Constant8 : Constant  Value=r_S
  Constant9 : Constant  Value=I_S
  inertiajoint_fcn : MATLAB Function  TreatAsAtomicUnit=on
  Mq : Outport  PortDimensions=[6+NQJ 6+NQJ]
  wires:
  inertiajoint_fcn/1(Mq) -> Mq/1
  Constant6/1 -> inertiajoint_fcn/3(pkin)
  qJ/1 -> inertiajoint_fcn/1(qJ)
  Constant7/1 -> inertiajoint_fcn/4(m)
  Constant8/1 -> inertiajoint_fcn/5(r_S)
  Constant9/1 -> inertiajoint_fcn/6(I_S)
  phi_base/1 -> inertiajoint_fcn/2(phi_base)

== matlab function S7RRRRRRR1_coriolisvec_fixb_mp/coriolisvec_fcn ==
  data: q input double; taug output double; qD input double; pkin input double; MPV input double
function taug = coriolis(q, qD, pkin, MPV)
%#codegen
tauc_reg = S7RRRRRRR1_coriolisvecJ_fixb_regmin_slag_vp(q, qD, pkin);
taug = tauc_reg*MPV;

== matlab function S7RRRRRRR1_gravload_mp/gravload_Fcn ==
  data: q input double; taug output double; g_base input double; pkin input double; MPV input double
function taug = gravload(q, g_base, pkin, MPV)
%#codegen
taug_reg = S7RRRRRRR1_gravloadJ_regmin_slag_vp(q, g_base, pkin);
taug = taug_reg*MPV;

== matlab function S7RRRRRRR1_inertiaJ_mp/inertia_fcn ==
  data: q input double; Mq output double; pkin input double; MPV input double
function Mq = inertia(q, pkin, MPV)
%#codegen
Mq_reg = S7RRRRRRR1_inertiaJ_regmin_slag_vp(q, pkin);
Mq_mpv_vec = Mq_reg*MPV;
Mq = vec2symmat(Mq_mpv_vec);

== matlab function S7RRRRRRR1_energykin_fixb_mp/energykin_fcn ==
  data: q input double; T output double; qD input double; pkin input double; MPV input double
function T = energykin(q, qD, pkin, MPV)
%#codegen
t_reg = S7RRRRRRR1_energykin_fixb_regmin_slag_vp(q, qD, pkin);
T = t_reg*MPV;

== matlab function S7RRRRRRR1_energypot_fixb_mp/energypot_fcn ==
  data: q input double; T output double; g_base input double; pkin input double; MPV input double
function T = energypot(q, g_base, pkin, MPV)
%#codegen
t_reg = S7RRRRRRR1_energypot_fixb_regmin_slag_vp(q, g_base, pkin);
T = t_reg*MPV;

== matlab function S7RRRRRRR1_gravload_vp1/MATLAB Function ==
  data: q input double; taug output double; g_base input double; pkin input double; m input double; r_S input double
function taug = gravload(q, g_base, pkin, m, r_S)
%#codegen
taug = S7RRRRRRR1_gravloadJ_floatb_twist_slag_vp1(q, g_base, pkin, m, r_S);

== matlab function S7RRRRRRR1_coriolisvec_fixb_vp1/coriolisvec_fcn ==
  data: q input double; tauc output double; qD input double; pkin input double; m input double; r_S input double; I_S input double
function tauc = coriolis(q, qD, pkin, m, r_S, I_S)
%#codegen
tauc = S7RRRRRRR1_coriolisvecJ_fixb_slag_vp1(q, qD, pkin, m, r_S, I_S);

== matlab function S7RRRRRRR1_inertiaJ_vp1/inertiajoint_fcn ==
  data: q input double; Mq output double; pkin input double; m input double; r_S input double; I_S input double
function Mq = inertia(q, pkin, m, r_S, I_S)
%#codegen
Mq = S7RRRRRRR1_inertiaJ_slag_vp1(q, pkin, m, r_S, I_S);

== matlab function S7RRRRRRR1_energykin_fixb_vp1/MATLAB Function ==
  data: q input double; T output double; qD input double; pkin input double; m input double; r_S input double; I_S input double
function T = energykin(q, qD, pkin, m, r_S, I_S)
%#codegen
T = S7RRRRRRR1_energykin_fixb_slag_vp1(q, qD, pkin, m, r_S, I_S);

== matlab function S7RRRRRRR1_energypot_fixb_vp1/MATLAB Function ==
  data: q input double; U output double; g_base input double; pkin input double; m input double; r_S input double
function U = energypot(q, g_base, pkin, m, r_S)
%#codegen
U = S7RRRRRRR1_energypot_fixb_slag_vp1(q, g_base, pkin, m, r_S);

== matlab function S7RRRRRRR1_fordyn_fixb_vp1/mFcn_Minv ==
  data: M input double; q_ddot output double; tau input double
function q_ddot = fcn(M,tau)
%#codegen
q_ddot=M\tau;

== matlab function S7RRRRRRR1_gravload_floatb_eulxyz_vp1/MATLAB Function ==
  data: q input double; taug output double; ob input double; g_world input double; pkin input double; m input double; r_S input double
function taug = gravload(q, ob, g_world, pkin, m, r_S)
%#codegen

taug_base = S7RRRRRRR1_gravloadB_floatb_eulxyz_slag_vp1(q, ob, g_world, ...
  pkin, m, r_S);
taug_joints = S7RRRRRRR1_gravloadJ_floatb_eulxyz_slag_vp1(q, ob, g_world,...
  pkin, m, r_S);
taug = [taug_base; taug_joints];

== matlab function S7RRRRRRR1_coriolisvec_floatb_eulxyz_vp1/coriolisvec_fcn ==
  data: qJ input double; tauc output double; qJD input double; phi_base input double; xD_base input double; pkin input double; m input double; r_S input double; I_S input double
function tauc = coriolis(qJ, qJD, phi_base, xD_base, pkin, m, r_S, I_S)
%#codegen
tauc = S7RRRRRRR1_coriolisvec_floatb_eulxyz_slag_vp1(qJ, qJD, phi_base, xD_base, ...
  pkin, m, r_S, I_S);

== matlab function S7RRRRRRR1_inertia_floatb_eulxyz_vp1/inertiajoint_fcn ==
  data: qJ input double; phi_base input double; Mq output double; pkin input double; m input double; r_S input double; I_S input double
function Mq = inertia(qJ, phi_base, pkin, m, r_S, I_S)
%#codegen
Mq = S7RRRRRRR1_inertia_floatb_eulxyz_slag_vp1(qJ, phi_base, ...
  pkin, m, r_S, I_S);

== matlab function S7RRRRRRR1_energypot_floatb_eulxyz_vp1/MATLAB Function ==
  data: qJ input double; U output double; r_base input double; phi_base input double; g_world input double; pkin input double; m input double; r_S input double
function U = energypot(qJ, r_base, phi_base, g_world, ...
  pkin, m, r_S)
%#codegen
U = S7RRRRRRR1_energypot_floatb_eulxyz_slag_vp1(qJ, r_base, phi_base, g_world, ...
  pkin, m, r_S);

== matlab function S7RRRRRRR1_energykin_floatb_eulxyz_vp1/MATLAB Function ==
  data: qJ input double; T output double; qD input double; phi_base input double; xD_base input double; pkin input double; m input double; r_S input double; I_S input double
function T = energykin(qJ, qD, phi_base, xD_base,  ...
  pkin, m, r_S, I_S)
%#codegen
T = S7RRRRRRR1_energykin_floatb_eulxyz_slag_vp1(qJ, qD, phi_base, xD_base, ...
  pkin, m, r_S, I_S);

== matlab function S7RRRRRRR1_gravload_floatb_eulxyz_mp/MATLAB Function ==
  data: q input double; taug output double; ob input double; g_world input double; pkin input double; MPV input double
function taug = gravload(q, ob, g_world, pkin, MPV)
%#codegen

tauBg_reg = S7RRRRRRR1_gravloadB_floatb_eulxyz_regmin_slag_vp(q, ob, g_world, pkin);
tauJg_reg = S7RRRRRRR1_gravloadJ_floatb_eulxyz_regmin_slag_vp(q, ob, g_world, pkin);    
taug_reg = [tauBg_reg;tauJg_reg];
taug = taug_reg*MPV;

== matlab function S7RRRRRRR1_coriolisvec_floatb_eulxyz_mp/coriolisvec_fcn ==
  data: qJ input double; tauc output double; qJD input double; phi_base input double; xD_base input double; pkin input double; MPV input double
function tauc = coriolis(qJ, qJD, phi_base, xD_base, pkin, MPV)
%#codegen
tauc_reg = S7RRRRRRR1_coriolisvec_floatb_eulxyz_regmin_slag_vp(qJ, qJD, ...
  phi_base, xD_base, pkin);

tauc = tauc_reg*MPV;

== matlab function S7RRRRRRR1_inertia_floatb_eulxyz_mp/inertiajoint_fcn ==
  data: qJ input double; phi_base input double; Mq output double; pkin input double; MPV input double
function Mq = inertia(qJ, phi_base, pkin, MPV)
%#codegen
M_regmin = S7RRRRRRR1_inertia_floatb_eulxyz_regmin_slag_vp(qJ, phi_base, pkin);
M_mpv_vec = M_regmin*MPV;
Mq = vec2symmat(M_mpv_vec);

== matlab function S7RRRRRRR1_energykin_floatb_eulxyz_mp/MATLAB Function ==
  data: qJ input double; T output double; qD input double; phi_base input double; xD_base input double; pkin input double; MPV input double
function T = energykin(qJ, qD, phi_base, xD_base,  ...
  pkin, MPV)
%#codegen
T_reg = S7RRRRRRR1_energykin_floatb_eulxyz_regmin_slag_vp(qJ, qD, phi_base, xD_base, ...
  pkin);

T = T_reg*MPV;

== matlab function S7RRRRRRR1_energypot_floatb_eulxyz_mp/MATLAB Function ==
  data: qJ input double; U output double; r_base input double; phi_base input double; g_world input double; pkin input double; MPV input double
function U = energypot(qJ, r_base, phi_base, g_world, ...
  pkin, MPV)
%#codegen
U_reg = S7RRRRRRR1_energypot_floatb_eulxyz_regmin_slag_vp(qJ, r_base, phi_base, g_world, ...
  pkin);
U = U_reg*MPV;

== matlab function S7RRRRRRR1_fordyn_floatb_eulxyz_mp/mFcn_Minv ==
  data: M input double; q_ddot output double; tau input double
function q_ddot = fcn(M,tau)
%#codegen
q_ddot=M\tau;

== matlab function S7RRRRRRR1_fordyn_floatb_eulxyz_vp1/mFcn_Minv ==
  data: M input double; q_ddot output double; tau input double
function q_ddot = fcn(M,tau)
%#codegen
q_ddot=M\tau;

== matlab function S7RRRRRRR1_fordyn_fixb_mp/mFcn_Minv ==
  data: M input double; q_ddot output double; tau input double
function q_ddot = fcn(M,tau)
%#codegen
q_ddot=M\tau;
